simulink model "problem18"  (R2018b)
settings: Solver=ode45  StartTime=0.0  StopTime=8  RelTol=1e-3  AbsTol=auo  EnableMultiTasking=on
values from neighbouring files (symbols this model uses):
  d1 = 1.6    [robotics_problem17.m]    (also in robotics_problem18.m; robotics_problem20.m; robotics_problem21.m; robotics_problem7.m = digits(32))
settings Model: Creator=Anders  LastModifiedBy=JanAriel
settings SolverCC: AutoScaleAbsTol=off
settings DataIOCC: LimitDataPoints=on  SaveFormat=Array  SignalLoggingSaveFormat=ModelDataLogs  SaveOutput=off  SaveTime=off  SignalLoggingName=sigsOut
settings OptimizationCC: ExpressionDepthLimit=2147483647  InitFltsAndDblsToZero=on  LifeSpan=inf
settings DebuggingCC: SaveWithParameterizedLinksMsg=none  UnderspecifiedInitializationDetection=Classic  MergeDetectMultiDrivingBlocksExec=none  SignalResolutionControl=TryResolveAllWithWarning  MultiTaskDSMMsg=warning  MultiTaskCondExecSysMsg=none  FcnCallInpInsideContextMsg=warning  StateNameClashWarn=warning  SFUnexpectedBacktrackingDiag=warning  SFNoUnconditionalDefaultTransitionDiag=warning  SFExecutionAtInitializationDiag=none
settings HardwareCC: ProdBitPerPointer=32  ProdBitPerSizeT=32  ProdBitPerPtrDiffT=32  ProdLargestAtomicFloat=None  ProdIntDivRoundTo=Undefined  ProdEndianess=Unspecified  ProdWordSize=32  ProdHWDeviceType=32-bit Generic  TargetUnknown=on
settings ModelReferenceCC: PropagateSignalLabelsOutOfModel=off
settings SFSimCC: SimUseLocalCustomCode=off
settings RTWCC: RTWUseLocalCustomCode=off
settings CodeAppCC: StateflowObjectComments=on
settings GRTTargetCC: TargetFcnLib=ansi_tfl_tmw.mat  TargetLangStandard=C89/C90 (ANSI)  GeneratePreprocessorConditionals=Disable all  CombineOutputUpdateFcns=off  GRTInterface=on
settings ConfigComp: CovMetricSettings=dw  CovHtmlReporting=on  CovSaveCumulativeToWorkspaceVar=on  CovSaveSingleToWorkspaceVar=on  CovExternalEMLEnable=off

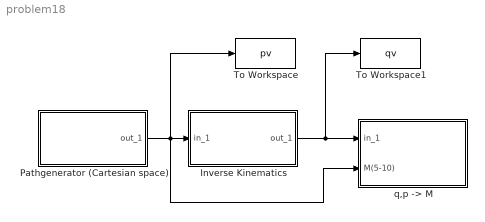
== system problem18 ==
  Inverse Kinematics : Subsystem
      mask Display: disp('Alto-Robot')
  "Pathgenerator (Cartesian space) " : Subsystem
      mask Display: disp('Alto-Robot\nPath -> p')
  To Workspace : ToWorkspace  VariableName=pv  SaveFormat=Structure With Time  SampleTime=-1
  To Workspace1 : ToWorkspace  VariableName=qv  SaveFormat=Structure With Time  SampleTime=-1
  "q,p -> M" : Subsystem
      mask Display: disp('Save to vis4link')
  wires:
  "Pathgenerator (Cartesian space) "/1(out_1) -> "q,p -> M"/2(M(5-10)), To Workspace/1, Inverse Kinematics/1(in_1)
  Inverse Kinematics/1(out_1) -> To Workspace1/1, "q,p -> M"/1(in_1)

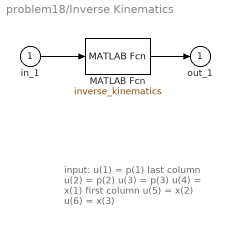
== system problem18/Inverse Kinematics ==
  note: input:
      | u(1) = p(1) last column
      | u(2) = p(2)
      | u(3) = p(3)
      | u(4) = x(1) first column
      | u(5) = x(2)
      | u(6) = x(3)
  in_1 : Inport
  MATLAB Fcn : MATLABFcn  MATLABFcn=inverse_kinematics  OutputDimensions=4
  out_1 : Outport
  wires:
  MATLAB Fcn/1 -> out_1/1
  in_1/1 -> MATLAB Fcn/1

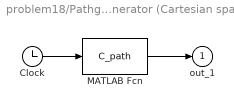
== system problem18/Pathgenerator (Cartesian space)  ==
  Clock : Clock
  MATLAB Fcn : MATLABFcn  MATLABFcn=C_path  OutputDimensions=6
  out_1 : Outport
  wires:
  Clock/1 -> MATLAB Fcn/1
  MATLAB Fcn/1 -> out_1/1

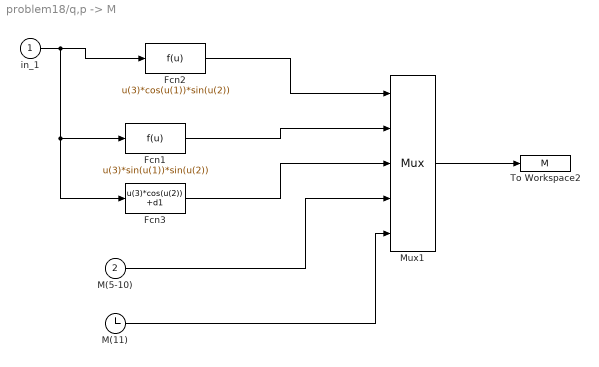
== system problem18/q,p -> M ==
  in_1 : Inport
  M(5-10) : Inport  Port=2
  Fcn1 : Fcn  Expr=u(3)*sin(u(1))*sin(u(2))
  Fcn2 : Fcn  Expr=u(3)*cos(u(1))*sin(u(2))
  Fcn3 : Fcn  Expr=u(3)*cos(u(2)) +d1
  M(11) : Clock
  Mux1 : Mux  Inputs=[1 1 1 6 1]
  To Workspace2 : ToWorkspace  VariableName=M
      settings: MaxDataPoints=100000
  wires:
  M(11)/1 -> Mux1/5
  M(5-10)/1 -> Mux1/4
  Fcn3/1 -> Mux1/3
  Fcn1/1 -> Mux1/2
  Fcn2/1 -> Mux1/1
  in_1/1 -> Fcn3/1, Fcn1/1, Fcn2/1
  Mux1/1 -> To Workspace2/1
